simulink model "SpeedControlModel"  (R2024b)
settings: Solver=VariableStepAuto  StartTime=0.0  StopTime=100  RelTol=1e-3
libraries: slpidlib x1
settings Model: Creator=amitl  LastModifiedBy=amitl

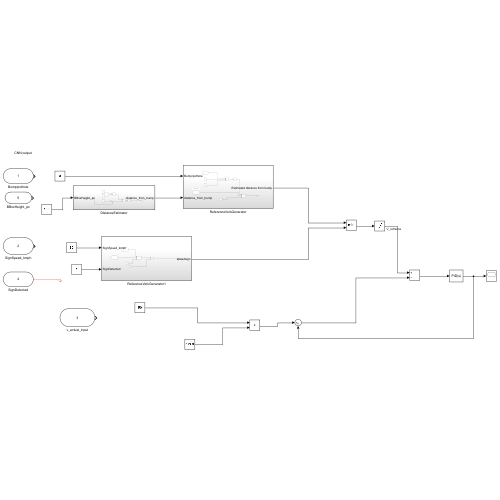
[thumbnail: Simulink's stored preview of the top-level diagram]
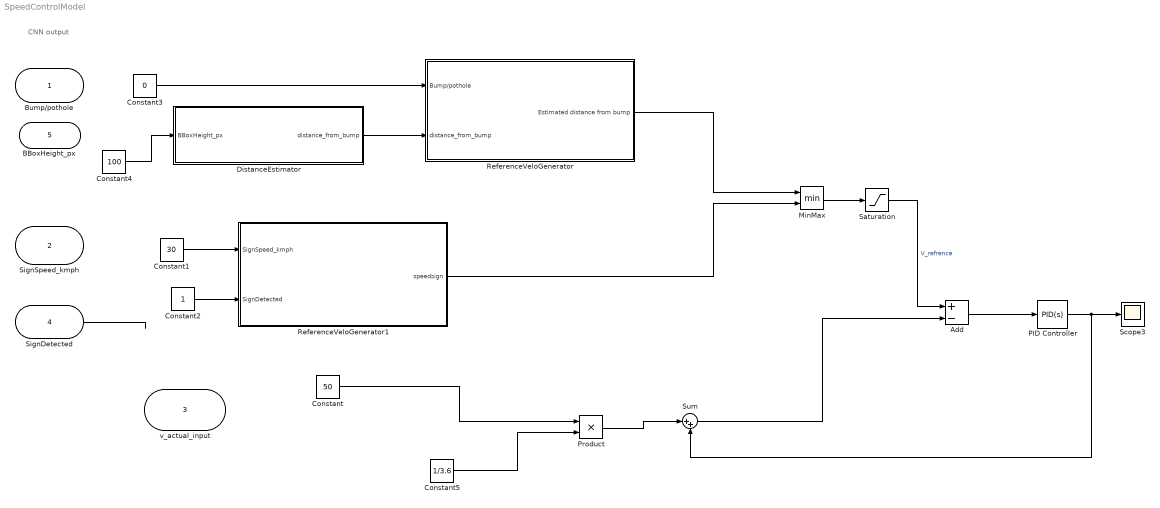
== system SpeedControlModel ==
  note: CNN output
  Bump/pothole : Inport
  SignSpeed_kmph : Inport  Port=2
  v_actual_input : Inport  Port=3
  SignDetected : Inport  Port=4
  BBoxHeight_px : Inport  Port=5
  Add : Sum  Inputs=+-
  Constant : Constant  Value=50
  Constant1 : Constant  Value=30
  Constant2 : Constant
  Constant3 : Constant  Value=0
  Constant4 : Constant  Value=100
  Constant5 : Constant  Value=1/3.6
  DistanceEstimator : Subsystem
  MinMax : MinMax  Inputs=2
  PID Controller : slpidlib/PID Controller  Controller=PID  Form=Parallel  TimeDomain=Continuous-time  UseExternalTs=off  SampleTime=-1  IntegratorMethod=Forward Euler  FilterMethod=Forward Euler  ControllerParametersSource=internal  P=200  I=1  UseKiTs=off  D=10  UseExternalDerivativeSource=off  N=100  UseFilter=on  TunerSelectOption=Transfer Function Based (PID Tuner App)  InitialConditionSource=internal  InitialConditionForIntegrator=0  InitialConditionForFilter=0  DifferentiatorICPrevScaledInput=0  ExternalReset=none  TrackingMode=off  Kt=1  LimitOutput=off  SatLimitsSource=internal  UpperSaturationLimit=inf  LowerSaturationLimit=-inf  LinearizeAsGain=on  AntiWindupMode=none  Kb=1  LimitIntegrator=off  UpperIntegratorSaturationLimit=inf  LowerIntegratorSaturationLimit=-inf  POutMin=[]  POutMax=[]  IOutMin=[]  IOutMax=[]  DOutMin=[]  DOutMax=[]  NOutMin=[]  NOutMax=[]  SumOutMin=[]  SumOutMax=[]  SaturationOutMin=[]  SaturationOutMax=[]  PParamMin=[]  PParamMax=[]  IParamMin=[]  IParamMax=[]  DParamMin=[]  DParamMax=[]  NParamMin=[]  NParamMax=[]  KbParamMin=[]  KbParamMax=[]  KtParamMin=[]  KtParamMax=[]  KbOutMin=[]  KbOutMax=[]  KtOutMin=[]  KtOutMax=[]  IntegratorOutMin=[]  IntegratorOutMax=[]  FilterOutMin=[]  FilterOutMax=[]  SumI1OutMin=[]  SumI1OutMax=[]  SumI2OutMin=[]  SumI2OutMax=[]  SumI3OutMin=[]  SumI3OutMax=[]  SumI4OutMin=[]  SumI4OutMax=[]  SumDOutMin=[]  SumDOutMax=[]  DifferentiatorOutMin=[]  DifferentiatorOutMax=[]  FilterDiffOutCoefMin=[]  FilterDiffOutCoefMax=[]  ReciprocalOutMin=[]  ReciprocalOutMax=[]  SumDenOutMin=[]  SumDenOutMax=[]  SumNumOutMin=[]  SumNumOutMax=[]  DivideOutMin=[]  DivideOutMax=[]  UdiffTsProdOutMin=[]  UdiffTsProdOutMax=[]  NTsProdOutMin=[]  NTsProdOutMax=[]  UintegralTsProdOutMin=[]  UintegralTsProdOutMax=[]  UngainTsProdOutMin=[]  UngainTsProdOutMax=[]  ClampingZeroOutDataTypeStr=Inherit: Inherit via back propagation  ClampingZeroOutMin=[]  ClampingZeroOutMax=[]  FilterDenConstantOutDataTypeStr=Inherit: Inherit via back propagation  FilterDenConstantOutMin=[]  FilterDenConstantOutMax=[]  PCopyOutDataTypeStr=Inherit: Inherit via back propagation  PCopyOutMin=[]  PCopyOutMax=[]  NCopyOutDataTypeStr=Inherit: Inherit via back propagation  NCopyOutMin=[]  NCopyOutMax=[]  IntegratorContinuousStateAttributes=''  IntegratorStateMustResolveToSignalObject=off  IntegratorRTWStateStorageClass=Auto  FilterContinuousStateAttributes=''  FilterStateMustResolveToSignalObject=off  FilterRTWStateStorageClass=Auto  ParallelPVariant=InternalParameters  IdealPVariant=Disabled  IVariant=InternalParameters  DVariant=InternalParameters  IntegratorVariant=Continuous  SatVariant=Disabled  AWVariant=Passthrough  PCopyVariant=Disabled  TRVariant=Disabled  FdbkBlocksVariant=Forward  IdealPFdbkVariant=Disabled  SatFdbkVariant=Disabled  DerivativeFilterVariant=ContFilter  NVariant=InternalParameters  NCopyVariant=Disabled  FilterICVariant=InternalICsFilter  IntegratorICVariant=InternalICs  ExternalResetVariant=Disabled  TRSumVariant=Passthrough  SumFdbkVariant=Disabled  SumVariant=Sum_PID  TsampFilterVariant=InternalTs  TsampNgainVariant=Passthrough  TsampIntegralVariant=Disabled_SignalSpec  ExternalSaturationOutDataTypeStr=Inherit: Same as second input  DerivativeSourceVariant=ErrorSignal  PreIntVariant=InternalPreInt
  Product : Product
  ReferenceVeloGenerator : Subsystem
  ReferenceVeloGenerator1 : Subsystem
  Saturation : Saturate  UpperLimit=40  LowerLimit=0
  Scope3 : Scope
  Sum : Sum  Inputs=|++
  wires:
  MinMax/1 -> Saturation/1
  Add/1 -> PID Controller/1
  ReferenceVeloGenerator/1(Estimated distance from bump) -> MinMax/1
  ReferenceVeloGenerator1/1(speedsign) -> MinMax/2
  DistanceEstimator/1(distance_from_bump) -> ReferenceVeloGenerator/2(distance_from_bump)
  SignDetected/1 -> ?
  Constant1/1 -> ReferenceVeloGenerator1/1(SignSpeed_kmph)
  Constant2/1 -> ReferenceVeloGenerator1/2(SignDetected)
  Constant4/1 -> DistanceEstimator/1(BBoxHeight_px)
  Constant3/1 -> ReferenceVeloGenerator/1(Bump/pothole)
  PID Controller/1 -> Sum/2, Scope3/1
  Sum/1 -> Add/2
  Constant/1 -> Product/1
  Saturation/1 -> Add/1  "V_refrence"
  Product/1 -> Sum/1
  Constant5/1 -> Product/2

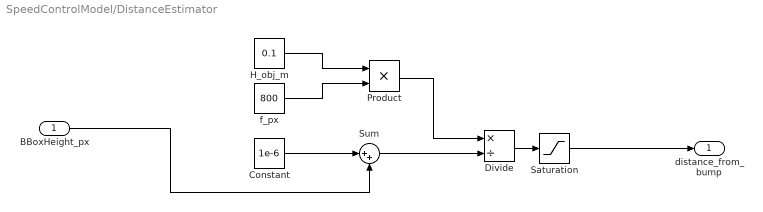
== system SpeedControlModel/DistanceEstimator ==
  BBoxHeight_px : Inport
  Constant : Constant  Value=1e-6
  Divide : Product  Inputs=*/
  H_obj_m : Constant  Value=0.1
  Product : Product
  Saturation : Saturate  UpperLimit=100  LowerLimit=0.05
  Sum : Sum  Inputs=|++
  f_px : Constant  Value=800
  distance_from_bump : Outport
  wires:
  Saturation/1 -> distance_from_bump/1
  f_px/1 -> Product/2
  Product/1 -> Divide/1
  Divide/1 -> Saturation/1
  BBoxHeight_px/1 -> Sum/2
  H_obj_m/1 -> Product/1
  Constant/1 -> Sum/1
  Sum/1 -> Divide/2

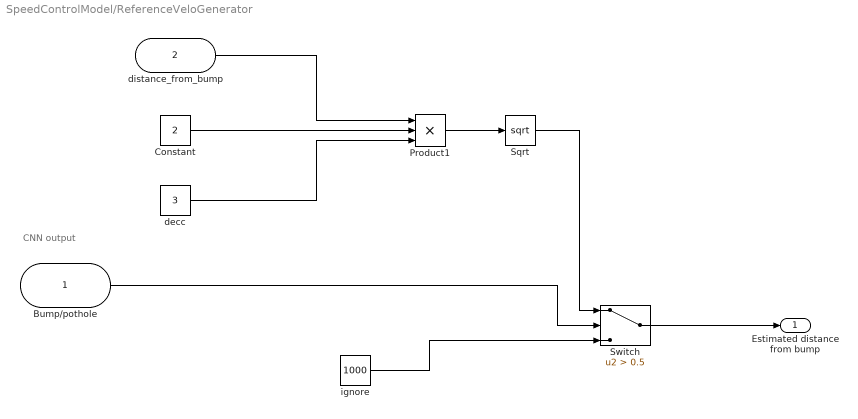
== system SpeedControlModel/ReferenceVeloGenerator ==
  note: CNN output
  Bump/pothole : Inport
  distance_from_bump : Inport  Port=2
  Constant : Constant  Value=2
  Product1 : Product  Inputs=3
  Sqrt : Sqrt
  Switch : Switch  Criteria=u2 > Threshold  Threshold=0.5  SaturateOnIntegerOverflow=off  InputSameDT=off
  decc : Constant  Value=3
  ignore : Constant  Value=1000
  Estimated distance from bump : Outport
  wires:
  decc/1 -> Product1/3
  Product1/1 -> Sqrt/1
  distance_from_bump/1 -> Product1/1
  Bump/pothole/1 -> Switch/2
  Constant/1 -> Product1/2
  Switch/1 -> Estimated distance from bump/1
  Sqrt/1 -> Switch/1
  ignore/1 -> Switch/3

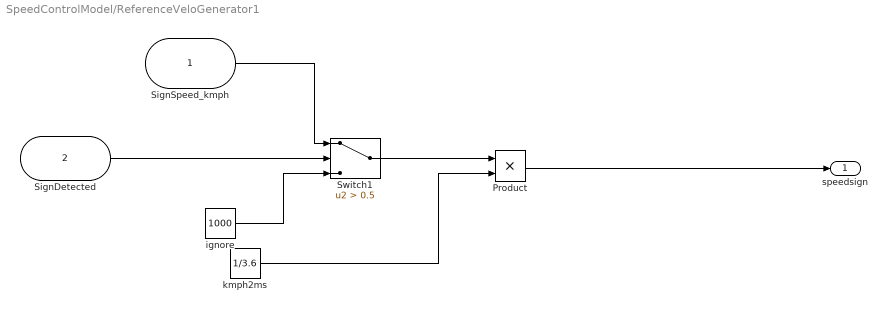
== system SpeedControlModel/ReferenceVeloGenerator1 ==
  SignSpeed_kmph : Inport
  SignDetected : Inport  Port=2
  Product : Product
  Switch1 : Switch  Criteria=u2 > Threshold  Threshold=0.5  SaturateOnIntegerOverflow=off  InputSameDT=off
  ignore : Constant  Value=1000
  kmph2ms : Constant  Value=1/3.6
  speedsign : Outport
  wires:
  Switch1/1 -> Product/1
  SignDetected/1 -> Switch1/2
  SignSpeed_kmph/1 -> Switch1/1
  kmph2ms/1 -> Product/2
  Product/1 -> speedsign/1
  ignore/1 -> Switch1/3
